simulink subsystem "DualArmStabilization"  (R2023a)
settings: Solver=VariableStepAuto  StartTime=0.0  StopTime=10.0  RelTol=1e-3
undefined symbols (not defined in the file or in its folder): arm, DiscIntNeverNeededParam, jointControlData
settings Model: Creator=Andy  LastModifiedBy=Andy
settings OptimizationCC: ReuseModelBlockBuffer=off
settings ModelReferenceCC: EnableRefExpFcnMdlSchedulingChecks=on

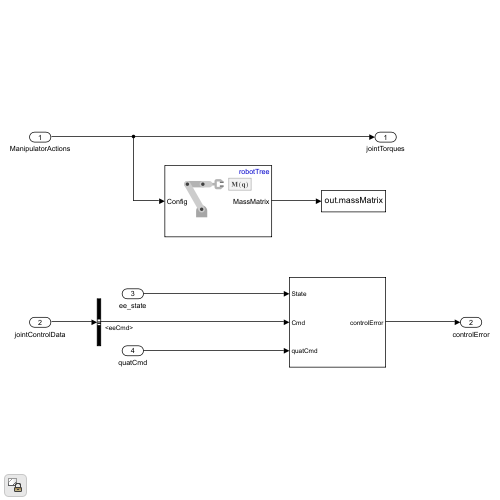
[thumbnail: Simulink's stored preview of the top-level diagram]
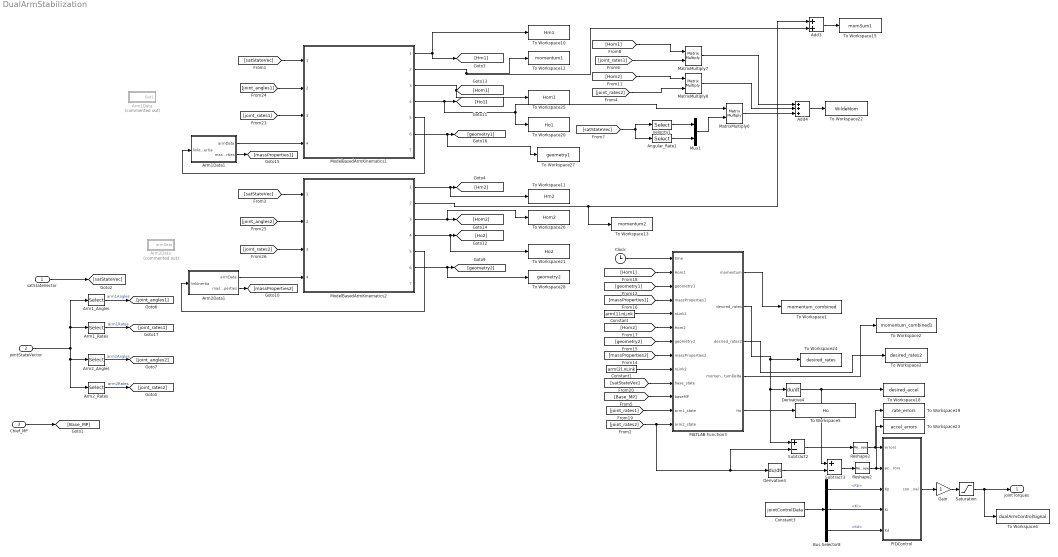
== system DualArmStabilization ==
  satStateVector : Inport
  jointStateVector : Inport  Port=2
  Chief_MP : Inport  Port=3
  Add3 : Sum
  Add4 : Sum  Inputs=+++
  Angular_Rate1 : Selector  InputPortWidth=12  IndexOptions=Index vector (dialog)  Indices=10:12  OutputSizes=1
  Arm1Data : Subsystem  Commented=on
  Arm1Data1 : Subsystem
  Arm1_Angles : Selector  IndexOptions=Index vector (dialog)  Indices=1:arm(1).nLink  OutputSizes=1
  Arm1_Rates : Selector  IndexOptions=Index vector (dialog)  Indices=1+arm(1).nLink+arm(2).nLink:2*arm(1).nLink+arm(2).nLink  OutputSizes=1
  Arm2Data : Subsystem  Commented=on
  Arm2Data1 : Subsystem
  Arm2_Angles : Selector  IndexOptions=Index vector (dialog)  Indices=1+arm(1).nLink:arm(1).nLink+arm(2).nLink  OutputSizes=1
  Arm2_Rates : Selector  IndexOptions=Index vector (dialog)  Indices=1+2*arm(1).nLink+arm(2).nLink:2*arm(1).nLink+2*arm(2).nLink  OutputSizes=1
  Bus Selector8 : BusSelector  OutputSignals=Kp,Ki,Kd
  Clock : Clock
  Constant : Constant  Value=arm(1).nLink
  Constant1 : Constant  Value=arm(2).nLink
  Constant3 : Constant  Value=jointControlData  OutDataTypeStr=Bus:jointControlDataBus
  Derivative3 : Derivative
  Derivative4 : Derivative
  Gain : Gain
  MATLAB Function3 : MATLAB Function  TreatAsAtomicUnit=on
  MatrixMultiply6 : Product  Multiplication=Matrix(*)
  MatrixMultiply7 : Product  Multiplication=Matrix(*)
  MatrixMultiply8 : Product  Multiplication=Matrix(*)
  ModelBasedArmKinematics1 : Subsystem  VariantControl=VSS_ModelBasedArmControl  ReferencedSubsystem=ModelBasedArmKinematics
  ModelBasedArmKinematics2 : Subsystem  VariantControl=VSS_ModelBasedArmControl  ReferencedSubsystem=ModelBasedArmKinematics
  Mux1 : Mux  Inputs=2
  PIDControl : Subsystem
  Reshape2 : Reshape  OutputDimensionality=Row vector (2-D)
  Reshape3 : Reshape  OutputDimensionality=Row vector (2-D)
  Saturation : Saturate  UpperLimit=jointControlData.torqueLimit  LowerLimit=-jointControlData.torqueLimit
  Subtract2 : Sum  Inputs=+-
  Subtract3 : Sum  Inputs=+-
  To Workspace1 : ToWorkspace  VariableName=momentum_combined  SaveFormat=Timeseries  SampleTime=-1
  To Workspace10 : ToWorkspace  VariableName=Hm1  SaveFormat=Timeseries  SampleTime=-1
  To Workspace11 : ToWorkspace  VariableName=Hm2  SaveFormat=Timeseries  SampleTime=-1
  To Workspace12 : ToWorkspace  VariableName=momentum1  SaveFormat=Timeseries  SampleTime=-1
  To Workspace13 : ToWorkspace  VariableName=momentum2  SaveFormat=Timeseries  SampleTime=-1
  To Workspace15 : ToWorkspace  VariableName=momSum1  SaveFormat=Timeseries  SampleTime=-1
  To Workspace18 : ToWorkspace  VariableName=desired_accel  SaveFormat=Timeseries  SampleTime=-1
  To Workspace19 : ToWorkspace  VariableName=rate_errors  SaveFormat=Timeseries  SampleTime=-1
  To Workspace2 : ToWorkspace  VariableName=momentum_combined1  SaveFormat=Timeseries  SampleTime=-1
  To Workspace20 : ToWorkspace  VariableName=Ho1  SaveFormat=Timeseries  SampleTime=-1
  To Workspace21 : ToWorkspace  VariableName=Ho2  SaveFormat=Timeseries  SampleTime=-1
  To Workspace22 : ToWorkspace  VariableName=WildeMom  SaveFormat=Timeseries  SampleTime=-1
  To Workspace23 : ToWorkspace  VariableName=accel_errors  SaveFormat=Timeseries  SampleTime=-1
  To Workspace24 : ToWorkspace  VariableName=desired_rates  SaveFormat=Timeseries  SampleTime=-1
  To Workspace25 : ToWorkspace  VariableName=Hom1  SaveFormat=Timeseries  SampleTime=-1
  To Workspace26 : ToWorkspace  VariableName=Hom2  SaveFormat=Timeseries  SampleTime=-1
  To Workspace27 : ToWorkspace  VariableName=geometry1  SaveFormat=Timeseries  SampleTime=-1
  To Workspace28 : ToWorkspace  VariableName=geometry2  SaveFormat=Timeseries  SampleTime=-1
  To Workspace3 : ToWorkspace  VariableName=desired_rates2  SaveFormat=Timeseries  SampleTime=-1
  To Workspace4 : ToWorkspace  VariableName=dualArmControlSignal  SaveFormat=Timeseries  SampleTime=-1
  To Workspace5 : ToWorkspace  VariableName=Ho  SaveFormat=Timeseries  SampleTime=-1
  Velocity1 : Selector  InputPortWidth=12  IndexOptions=Index vector (dialog)  Indices=7:9  OutputSizes=1
  jointTorques : Outport
  wires:
  Arm2_Rates/1 -> [joint_rates2]  "arm2Rates"
  Gain/1 -> Saturation/1
  jointStateVector/1 -> Arm2_Rates/1, Arm2_Angles/1, Arm1_Rates/1, Arm1_Angles/1
  Saturation/1 -> To Workspace4/1, jointTorques/1
  Arm1_Angles/1 -> [joint_angles1]  "arm1Angles"
  Arm1_Rates/1 -> [joint_rates1]  "arm1Rates"
  Arm2_Angles/1 -> [joint_angles2]  "arm2Angles"
  satStateVector/1 -> [satStateVec]
  [satStateVec] -> ModelBasedArmKinematics1/1
  [satStateVec] -> ModelBasedArmKinematics2/1
  ModelBasedArmKinematics1/1 -> To Workspace10/1, [Hm1]
  ModelBasedArmKinematics2/1 -> [Hm2], To Workspace11/1
  ModelBasedArmKinematics1/2 -> To Workspace12/1, Add3/2
  ModelBasedArmKinematics2/2 -> Add3/1, To Workspace13/1
  ModelBasedArmKinematics2/4 -> [Ho2], To Workspace21/1
  Add3/1 -> To Workspace15/1
  ModelBasedArmKinematics1/6 -> [geometry1], To Workspace27/1
  ModelBasedArmKinematics1/4 -> [Ho1], MatrixMultiply6/1, To Workspace20/1
  [satStateVec] -> Angular_Rate1/1, Velocity1/1
  Mux1/1 -> MatrixMultiply6/2
  Velocity1/1 -> Mux1/1
  Angular_Rate1/1 -> Mux1/2
  MatrixMultiply6/1 -> Add4/3
  ModelBasedArmKinematics1/3 -> [Hom1], To Workspace25/1
  ModelBasedArmKinematics2/3 -> [Hom2], To Workspace26/1
  [Hom1] -> MatrixMultiply7/1
  MatrixMultiply7/1 -> Add4/1
  [Hom2] -> MatrixMultiply8/1
  MatrixMultiply8/1 -> Add4/2
  Add4/1 -> To Workspace22/1
  [geometry1] -> MATLAB Function3/3(geometry1)
  [massProperties1] -> MATLAB Function3/4(massProperties1)
  [geometry2] -> MATLAB Function3/7(geometry2)
  [massProperties2] -> MATLAB Function3/8(massProperties2)
  [Hom2] -> MATLAB Function3/6(Hom2)
  Clock/1 -> MATLAB Function3/1(time)
  [Hom1] -> MATLAB Function3/2(Hom1)
  Derivative3/1 -> Subtract3/2
  Subtract2/1 -> Reshape3/1
  MATLAB Function3/2(desired_rates) -> To Workspace24/1, Derivative4/1, Subtract2/1
  Derivative4/1 -> To Workspace18/1, Subtract3/1
  Bus Selector8/2 -> PIDControl/4(Ki)  "<Ki>"
  Bus Selector8/1 -> PIDControl/3(Kp)  "<Kp>"
  Constant3/1 -> Bus Selector8/1
  Bus Selector8/3 -> PIDControl/5(Kd)  "<Kd>"
  Subtract3/1 -> Reshape2/1
  PIDControl/1(controlSignal) -> Gain/1
  [satStateVec] -> MATLAB Function3/10(base_state)
  Reshape2/1 -> PIDControl/2(accelErrors), To Workspace23/1
  Reshape3/1 -> PIDControl/1(errors), To Workspace19/1
  ModelBasedArmKinematics2/6 -> [geometry2], To Workspace28/1
  [joint_angles1] -> ModelBasedArmKinematics1/2
  [joint_rates1] -> ModelBasedArmKinematics1/3
  [joint_angles2] -> ModelBasedArmKinematics2/2
  [joint_rates2] -> ModelBasedArmKinematics2/3
  [joint_rates2] -> MATLAB Function3/13(arm2_state), Derivative3/1, Subtract2/2
  [joint_rates1] -> MATLAB Function3/12(arm1_state)
  [joint_rates2] -> MatrixMultiply8/2
  [joint_rates1] -> MatrixMultiply7/2
  Constant1/1 -> MATLAB Function3/9(nLink2)
  Constant/1 -> MATLAB Function3/5(nLink1)
  MATLAB Function3/1(momentum) -> To Workspace1/1
  Arm1Data1/1(armData) -> ModelBasedArmKinematics1/4
  Arm1Data1/2(massProperties) -> [massProperties1]
  ModelBasedArmKinematics1/5 -> Arm1Data1/1(linkInertia)
  Arm2Data1/1(armData) -> ModelBasedArmKinematics2/4
  ModelBasedArmKinematics2/5 -> Arm2Data1/1(linkInertia)
  Arm2Data1/2(massProperties) -> [massProperties2]
  [Base_MP] -> MATLAB Function3/11(baseMP)
  Chief_MP/1 -> [Base_MP]
  MATLAB Function3/4(momentumDelta) -> To Workspace2/1
  MATLAB Function3/3(desired_rates2) -> To Workspace3/1
  MATLAB Function3/5(Ho) -> To Workspace5/1

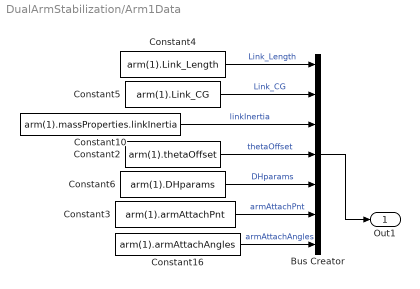
== system DualArmStabilization/Arm1Data ==
  Bus Creator : BusCreator  Inputs=7
  Constant10 : Constant  Value=arm(1).massProperties.linkInertia
  Constant16 : Constant  Value=arm(1).armAttachAngles
  Constant2 : Constant  Value=arm(1).thetaOffset
  Constant3 : Constant  Value=arm(1).armAttachPnt
  Constant4 : Constant  Value=arm(1).Link_Length
  Constant5 : Constant  Value=arm(1).Link_CG
  Constant6 : Constant  Value=arm(1).DHparams
  Out1 : Outport
  wires:
  Constant2/1 -> Bus Creator/4  "thetaOffset"
  Constant6/1 -> Bus Creator/5  "DHparams"
  Constant10/1 -> Bus Creator/3  "linkInertia"
  Constant5/1 -> Bus Creator/2  "Link_CG"
  Constant4/1 -> Bus Creator/1  "Link_Length"
  Constant3/1 -> Bus Creator/6  "armAttachPnt"
  Constant16/1 -> Bus Creator/7  "armAttachAngles"
  Bus Creator/1 -> Out1/1

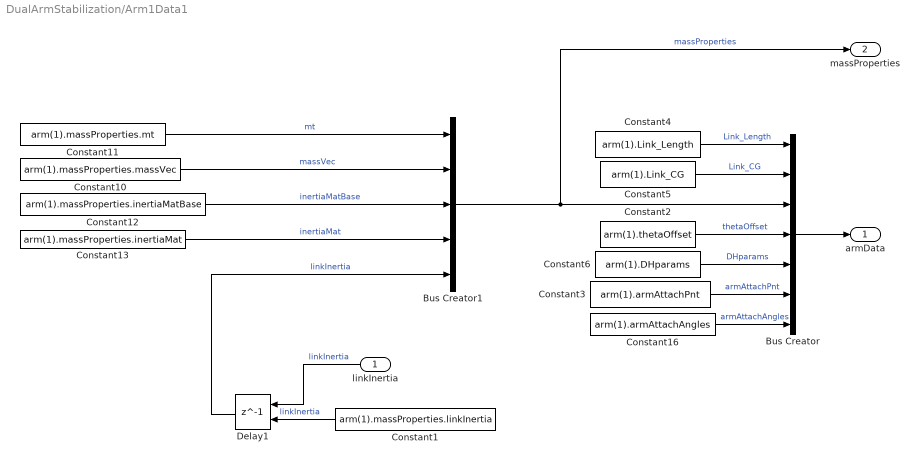
== system DualArmStabilization/Arm1Data1 ==
  linkInertia : Inport
  Bus Creator : BusCreator  Inputs=7
  Bus Creator1 : BusCreator  Inputs=5  OutDataTypeStr=Bus: MassPropertiesBus
      settings: InheritFromInputs=off
  Constant1 : Constant  Value=arm(1).massProperties.linkInertia
  Constant10 : Constant  Value=arm(1).massProperties.massVec
  Constant11 : Constant  Value=arm(1).massProperties.mt
  Constant12 : Constant  Value=arm(1).massProperties.inertiaMatBase
  Constant13 : Constant  Value=arm(1).massProperties.inertiaMat
  Constant16 : Constant  Value=arm(1).armAttachAngles
  Constant2 : Constant  Value=arm(1).thetaOffset
  Constant3 : Constant  Value=arm(1).armAttachPnt
  Constant4 : Constant  Value=arm(1).Link_Length
  Constant5 : Constant  Value=arm(1).Link_CG
  Constant6 : Constant  Value=arm(1).DHparams
  Delay1 : Delay  DelayLength=1  InitialConditionSource=Input port
      settings: InputPortMap=u0,p4
  armData : Outport
  massProperties : Outport  Port=2
  wires:
  linkInertia/1 -> Delay1/1  "linkInertia"
  Delay1/1 -> Bus Creator1/5  "linkInertia"
  Constant1/1 -> Delay1/2  "linkInertia"
  Bus Creator1/1 -> Bus Creator/3, massProperties/1  "massProperties"
  Constant11/1 -> Bus Creator1/1  "mt"
  Constant10/1 -> Bus Creator1/2  "massVec"
  Constant13/1 -> Bus Creator1/4  "inertiaMat"
  Constant12/1 -> Bus Creator1/3  "inertiaMatBase"
  Constant2/1 -> Bus Creator/4  "thetaOffset"
  Constant6/1 -> Bus Creator/5  "DHparams"
  Constant5/1 -> Bus Creator/2  "Link_CG"
  Constant4/1 -> Bus Creator/1  "Link_Length"
  Constant3/1 -> Bus Creator/6  "armAttachPnt"
  Constant16/1 -> Bus Creator/7  "armAttachAngles"
  Bus Creator/1 -> armData/1

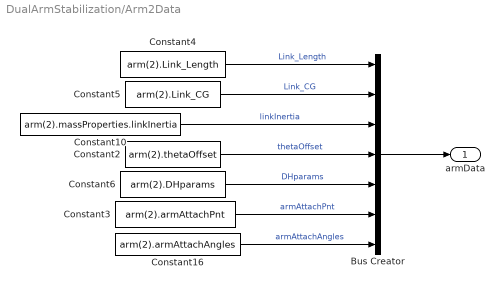
== system DualArmStabilization/Arm2Data ==
  Bus Creator : BusCreator  Inputs=7
  Constant10 : Constant  Value=arm(2).massProperties.linkInertia
  Constant16 : Constant  Value=arm(2).armAttachAngles
  Constant2 : Constant  Value=arm(2).thetaOffset
  Constant3 : Constant  Value=arm(2).armAttachPnt
  Constant4 : Constant  Value=arm(2).Link_Length
  Constant5 : Constant  Value=arm(2).Link_CG
  Constant6 : Constant  Value=arm(2).DHparams
  armData : Outport
  wires:
  Bus Creator/1 -> armData/1
  Constant16/1 -> Bus Creator/7  "armAttachAngles"
  Constant3/1 -> Bus Creator/6  "armAttachPnt"
  Constant4/1 -> Bus Creator/1  "Link_Length"
  Constant5/1 -> Bus Creator/2  "Link_CG"
  Constant10/1 -> Bus Creator/3  "linkInertia"
  Constant6/1 -> Bus Creator/5  "DHparams"
  Constant2/1 -> Bus Creator/4  "thetaOffset"

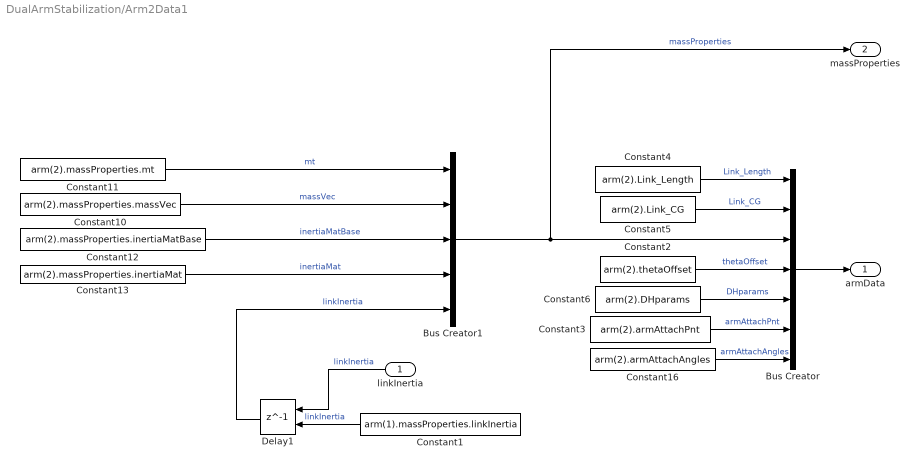
== system DualArmStabilization/Arm2Data1 ==
  linkInertia : Inport
  Bus Creator : BusCreator  Inputs=7
  Bus Creator1 : BusCreator  Inputs=5  OutDataTypeStr=Bus: MassPropertiesBus
      settings: InheritFromInputs=off
  Constant1 : Constant  Value=arm(1).massProperties.linkInertia
  Constant10 : Constant  Value=arm(2).massProperties.massVec
  Constant11 : Constant  Value=arm(2).massProperties.mt
  Constant12 : Constant  Value=arm(2).massProperties.inertiaMatBase
  Constant13 : Constant  Value=arm(2).massProperties.inertiaMat
  Constant16 : Constant  Value=arm(2).armAttachAngles
  Constant2 : Constant  Value=arm(2).thetaOffset
  Constant3 : Constant  Value=arm(2).armAttachPnt
  Constant4 : Constant  Value=arm(2).Link_Length
  Constant5 : Constant  Value=arm(2).Link_CG
  Constant6 : Constant  Value=arm(2).DHparams
  Delay1 : Delay  DelayLength=1  InitialConditionSource=Input port
      settings: InputPortMap=u0,p4
  armData : Outport
  massProperties : Outport  Port=2
  wires:
  Delay1/1 -> Bus Creator1/5  "linkInertia"
  Constant1/1 -> Delay1/2  "linkInertia"
  linkInertia/1 -> Delay1/1  "linkInertia"
  Bus Creator/1 -> armData/1
  Constant16/1 -> Bus Creator/7  "armAttachAngles"
  Constant3/1 -> Bus Creator/6  "armAttachPnt"
  Constant4/1 -> Bus Creator/1  "Link_Length"
  Constant5/1 -> Bus Creator/2  "Link_CG"
  Constant6/1 -> Bus Creator/5  "DHparams"
  Constant2/1 -> Bus Creator/4  "thetaOffset"
  Constant12/1 -> Bus Creator1/3  "inertiaMatBase"
  Constant13/1 -> Bus Creator1/4  "inertiaMat"
  Constant10/1 -> Bus Creator1/2  "massVec"
  Constant11/1 -> Bus Creator1/1  "mt"
  Bus Creator1/1 -> Bus Creator/3, massProperties/1  "massProperties"

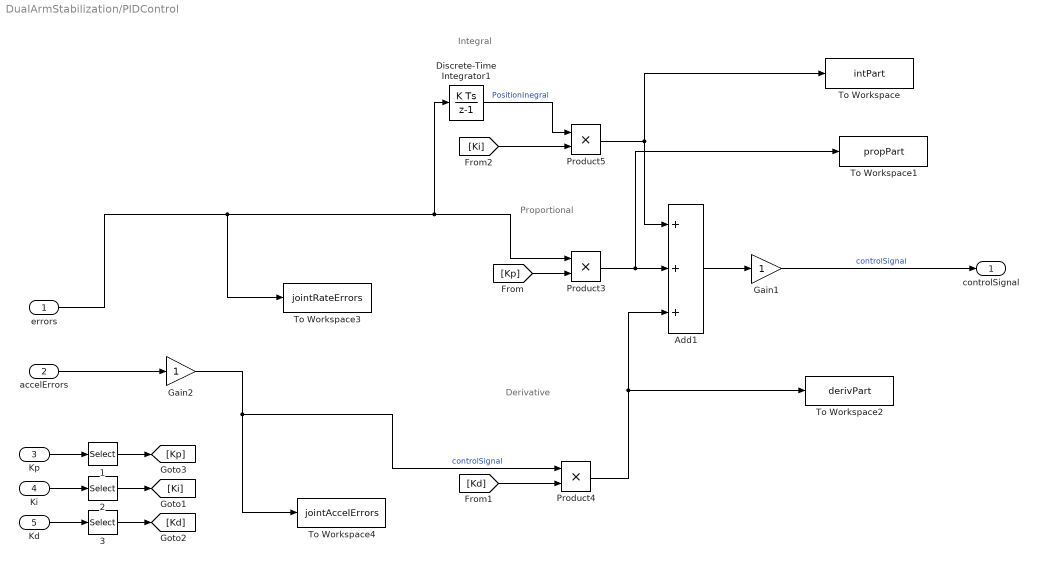
== system DualArmStabilization/PIDControl ==
  note: Integral
  note: Proportional
  note: Derivative
  errors : Inport
  accelErrors : Inport  Port=2
  Kp : Inport  Port=3
  Ki : Inport  Port=4
  Kd : Inport  Port=5
  1 : Selector  IndexOptions=Index vector (dialog)  Indices=1:arm(2).nLink  OutputSizes=1
  2 : Selector  IndexOptions=Index vector (dialog)  Indices=1:arm(2).nLink  OutputSizes=1
  3 : Selector  IndexOptions=Index vector (dialog)  Indices=1:arm(2).nLink  OutputSizes=1
  Add1 : Sum  Inputs=+++
  Discrete-Time Integrator1 : DiscreteIntegrator  SampleTime=-1  ICPrevOutput=DiscIntNeverNeededParam  ICPrevScaledInput=DiscIntNeverNeededParam
  Gain1 : Gain
  Gain2 : Gain
  Product3 : Product
  Product4 : Product
  Product5 : Product
  To Workspace : ToWorkspace  VariableName=intPart  SaveFormat=Timeseries  SampleTime=-1
  To Workspace1 : ToWorkspace  VariableName=propPart  SaveFormat=Timeseries  SampleTime=-1
  To Workspace2 : ToWorkspace  VariableName=derivPart  SaveFormat=Timeseries  SampleTime=-1
  To Workspace3 : ToWorkspace  VariableName=jointRateErrors  SaveFormat=Timeseries  SampleTime=-1
  To Workspace4 : ToWorkspace  VariableName=jointAccelErrors  SaveFormat=Timeseries  SampleTime=-1
  controlSignal : Outport
  wires:
  Gain2/1 -> Product4/1, To Workspace4/1  "controlSignal"
  accelErrors/1 -> Gain2/1
  3/1 -> [Kd]
  2/1 -> [Ki]
  1/1 -> [Kp]
  Product3/1 -> Add1/2, To Workspace1/1
  Ki/1 -> 2/1
  Kd/1 -> 3/1
  Kp/1 -> 1/1
  Product4/1 -> Add1/3, To Workspace2/1
  Add1/1 -> Gain1/1
  [Kd] -> Product4/2
  [Kp] -> Product3/2
  [Ki] -> Product5/2
  Gain1/1 -> controlSignal/1  "controlSignal"
  Product5/1 -> To Workspace/1, Add1/1
  Discrete-Time Integrator1/1 -> Product5/1  "PositionInegral"
  errors/1 -> Product3/1, Discrete-Time Integrator1/1, To Workspace3/1

== matlab function DualArmStabilization/MATLAB Function3 ==
  data: time input; Hom1 input; geometry1 input; momentum output; massProperties1 input; nLink1 input; Hom2 input; geometry2 input; massProperties2 input; nLink2 input; base_state input; baseMP input; arm1_state input; arm2_state input; desired_rates output; desired_rates2 output; momentumDelta output; Ho output
function [momentum,desired_rates,desired_rates2,momentumDelta,Ho] = calldualArmStabilizationControl(time,Hom1,geometry1,massProperties1,nLink1,Hom2,geometry2,massProperties2,nLink2,base_state,baseMP,arm1_state,arm2_state)
                                
%[momentum,desired_rates] = dualArmStabilizationControl(time,Hom1,geometry1,massProperties1,nLink1,Hom2,geometry2,massProperties2,nLink2,base_state,arm1_state,arm2_state);                                
[momentum,desired_rates,desired_rates2,momentumDelta,Ho] = dualArmStabilizationControl(time,Hom1,geometry1,massProperties1,nLink1,Hom2,geometry2,massProperties2,nLink2,base_state,baseMP,arm1_state,arm2_state);
